simulink model "sfcndemo_sfun_zc"  (Simulink 7.6)
settings: Solver=VariableStepDiscrete  StartTime=0.0  StopTime=10.0  RelTol=1e-3
Description:
  | Absolute Value Using Non-Sampled Zero Crossings C-MEX S-function
settings Model: Creator=The MathWorks Inc.  ExtModeTrigMode=oneshot  ExtModeArmWhenConnect=off  ExtModeAutoUpdateStatusClock=off
settings DataIOCC: LimitDataPoints=off
settings OptimizationCC: BlockReduction=off  BooleanDataType=off  InitFltsAndDblsToZero=on
settings DebuggingCC: SaveWithParameterizedLinksMsg=none  SignalResolutionControl=TryResolveAllWithWarning  SolverPrmCheckMsg=none  MultiTaskDSMMsg=warning  MultiTaskCondExecSysMsg=none
settings HardwareCC: TargetUnknown=on
settings RTWCC: TemplateMakefile=grt_vc.tmf  IncludeERTFirstTime=on
settings CodeAppCC: CustomSymbolStrFcn=$F$N$M
settings GRTTargetCC: TargetFcnLib=ansi_tfl_tmw.mat

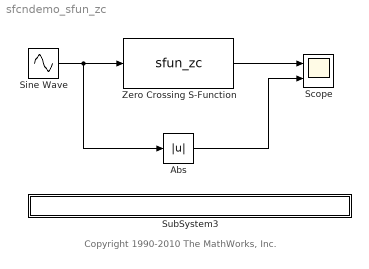
== system sfcndemo_sfun_zc ==
  note: Copyright 1990-2010 The MathWorks, Inc.
  Abs : Abs  SaturateOnIntegerOverflow=on
  Scope : Scope  NumInputPorts=2
      settings: TimeRange=10  YMin=0~0  YMax=2~2
  Sine Wave : Sin  Amplitude=1:2  SampleTime=0
  SubSystem3 : Subsystem  mask{filename=sfun_zc.c}
      mask init:
      | x=sfundemo_maskdisp;
      settings: AttributesFormatString=\n  OpenFcn=sfundemo_openfcn
      mask Display: disp(x);
  Zero Crossing S-Function : S-Function  FunctionName=sfun_zc  EnableBusSupport=off
      mask Type: S-function: sfun_zc
      mask Description: This is a S-function block which has nonsampled zero crossings.
  wires:
  Zero Crossing S-Function/1 -> Scope/1
  Abs/1 -> Scope/2
  Sine Wave/1 -> Zero Crossing S-Function/1, Abs/1

== system sfcndemo_sfun_zc/SubSystem3 ==
